simulink model "power_buckconv"  (Simulink 6.0)
settings: Solver=ode23tb  SolverMode=SingleTasking  StartTime=0.0  StopTime=0.01  RelTol=1e-3
libraries: powerlib x13
settings Model: Creator=patrice  LastModifiedBy=batserve  ExtModeTrigMode=oneshot  ExtModeArmWhenConnect=off  ExtModeAutoUpdateStatusClock=off
settings DataIOCC: LimitDataPoints=off  SignalLoggingName=sigsOut
settings OptimizationCC: BooleanDataType=off
settings DebuggingCC: SolverPrmCheckMsg=none
settings HardwareCC: TargetUnknown=on
settings RTWCC: TemplateMakefile=grt_unix.tmf

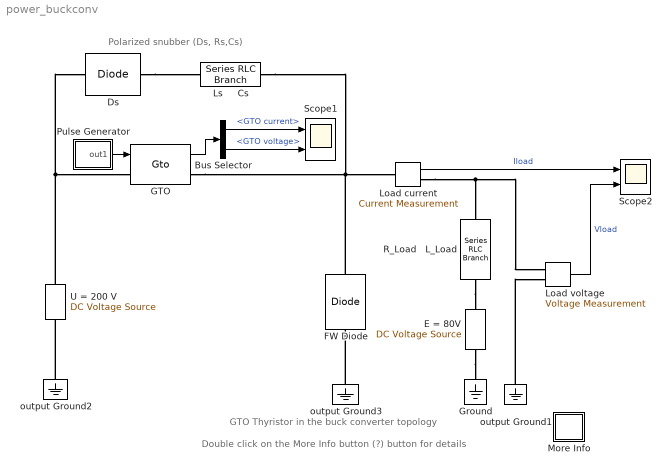
== system power_buckconv ==
  note: Double click on the More Info button (?) button for details
  note: GTO Thyristor in the buck converter topology
  note: Polarized snubber (Ds, Rs,Cs)
  Bus Selector : BusSelector  DialogController=Simulink.DDGSource_Bus  OutputSignals=GTO current,GTO voltage
  Ds : powerlib/Power Electronics/Diode  Ron=0.01  Lon=1e-6  Vf=0.8  IC=0  Rs=100  Cs=Inf  Measurements=off
  E = 80V : powerlib/Electrical Sources/DC Voltage Source  Description=source block  Orientation=up  Amplitude=80  Measurements=None
      settings: AttributesFormatString=\n
  FW Diode : powerlib/Power Electronics/Diode  Orientation=up  Ron=0.01  Lon=1e-6  Vf=0.8  IC=0  Rs=100  Cs=0.1e-6  Measurements=off
  GTO : powerlib/Power Electronics/Gto  Ron=0.01  Lon=1e-6  Vf=1  Tf=10e-6  Tt=20e-6  IC=0  Rs=Inf  Cs=0  Measurements=on
      settings: AttributesFormatString=\n
  Ground : powerlib/Elements/Ground  Orientation=down  PhysicalDomain=powersysdomain  SubClassName=unknown  LeftPortType=p1  RightPortType=p1  LConnTagsString=a
  Load current : powerlib/Measurements/Current Measurement  Tag=PoWeRsYsTeMmEaSuReMeNt  PhasorSimulation=off  OutputType=Magnitude  PSBequivalent=0
  Load voltage : powerlib/Measurements/Voltage Measurement  Tag=PoWeRsYsTeMmEaSuReMeNt  PhasorSimulation=off  OutputType=Magnitude  PSBequivalent=0
  Ls     Cs : powerlib/Elements/Series RLC Branch  PhysicalDomain=powersysdomain  SubClassName=unknown  LeftPortType=p1  RightPortType=p1  LConnTagsString=__new0  RConnTagsString=__new0  Resistance=0  Inductance=5e-7  Capacitance=2e-6  Measurements=None
  More Info : Subsystem
      mask Display: disp('?')
  Pulse Generator : Subsystem  mask(Pulse Generator){period=1e-3, duty=60, amplitude=1, start=0}
      mask prompts: period "Period (secs):"; duty "Duty cycle (% of period):"; start "Start time:"
      mask help: Pulse Generator
      mask Help: Pulse generator which ensures pulse transitions are hit. Provides a vector of pulses when the height is entered as a vector.  Unmask to see how it works.
      mask Display: plot(0,0,100,100,[95,90,90,75,75,60,60,45,45,30,30,15,15,5],[25,25,75,75,25,25,75,75,25,25,75,75,25,25]);
  R_Load   L_Load : powerlib/Elements/Series RLC Branch  Orientation=down  PhysicalDomain=powersysdomain  SubClassName=unknown  LeftPortType=p1  RightPortType=p1  LConnTagsString=__new0  RConnTagsString=__new0  Resistance=1  Inductance=5e-03  Capacitance=inf  Measurements=None
  Scope1 : Scope  NumInputPorts=2
      settings: TimeRange=0.01  YMin=-50~-100  YMax=50~200  DataFormat=Array  MaxDataPoints=500000
  Scope2 : Scope  NumInputPorts=2
      settings: TimeRange=0.01  YMin=-50~-100  YMax=50~200  DataFormat=Array  MaxDataPoints=500000
  U = 200 V : powerlib/Electrical Sources/DC Voltage Source  Description=source block  Orientation=up  Amplitude=200  Measurements=None
      settings: AttributesFormatString=\n
  output Ground1 : powerlib/Elements/Ground  Orientation=down  PhysicalDomain=powersysdomain  SubClassName=unknown  LeftPortType=p1  RightPortType=p1  LConnTagsString=a
  output Ground2 : powerlib/Elements/Ground  Orientation=down  PhysicalDomain=powersysdomain  SubClassName=unknown  LeftPortType=p1  RightPortType=p1  LConnTagsString=a
  output Ground3 : powerlib/Elements/Ground  Orientation=down  PhysicalDomain=powersysdomain  SubClassName=unknown  LeftPortType=p1  RightPortType=p1  LConnTagsString=a
  wires:
  Load current/1 -> Scope2/1  "Iload"
  Load voltage/1 -> Scope2/2  "Vload"
  GTO/1 -> Bus Selector/1
  Pulse Generator/1(out1) -> GTO/1
  Bus Selector/1 -> Scope1/1  "<GTO current>"
  Bus Selector/2 -> Scope1/2  "<GTO voltage>"
  connections:
  Ds/RConn1 -- Ls     Cs/LConn1
  Load current/RConn1 -- Load voltage/LConn1 -- R_Load   L_Load/LConn1
  output Ground1/LConn1 -- Load voltage/LConn2
  output Ground3/LConn1 -- FW Diode/LConn1
  E = 80V/LConn1 -- Ground/LConn1
  R_Load   L_Load/RConn1 -- E = 80V/RConn1
  U = 200 V/RConn1 -- GTO/LConn1 -- Ds/LConn1
  output Ground2/LConn1 -- U = 200 V/LConn1
  Ls     Cs/RConn1 -- FW Diode/RConn1 -- Load current/LConn1 -- GTO/RConn1

== system power_buckconv/More Info ==
  note: A basic polarized snubber circuit (consisting of Ds, Rs and Cs) is connected across the GTO.
      | The parasitic inductance Ls of the snubber is also taken into consideration.
      | The operating frequency is 1 kHz and the duty cycle is 60%.
  note: This example illustrates use of the GTO-thyristor in the buck converter topology
  note: Circuit Description

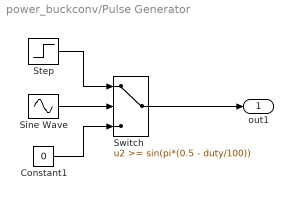
== system power_buckconv/Pulse Generator ==
  Constant1 : Constant  Value=0
  Sine Wave : Sin  Frequency=2*pi./period  Phase=-2*pi*(start./period + duty/200 - 1/4)  SampleTime=0
  Step : Step  Time=start  After=amplitude  SampleTime=0
  Switch : Switch  Threshold=sin(pi*(0.5 - duty/100))  SaturateOnIntegerOverflow=on  InputSameDT=on
  out1 : Outport  InitialOutput=0
  wires:
  Step/1 -> Switch/1
  Constant1/1 -> Switch/3
  Switch/1 -> out1/1
  Sine Wave/1 -> Switch/2
